simulink model "sun_path_1"  (R2017a)
settings: Solver=FixedStepAuto  StartTime=1  StopTime=1  FixedStep=1  RelTol=1e-3
libraries: simulink_extras x5
settings Model: Creator=zhiangz  LastModifiedBy=zhiangz

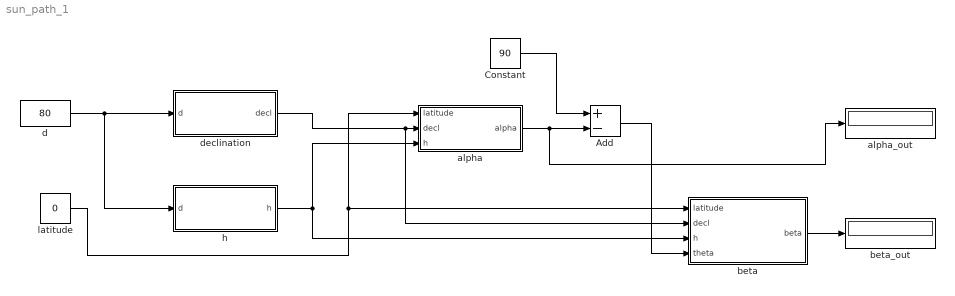
== system sun_path_1 ==
  Add : Sum  Inputs=+-
  Constant : Constant  Value=90
  alpha : Subsystem
  alpha_out : Display
  beta : Subsystem
  beta_out : Display
  d : Constant  Value=80
  declination : Subsystem
  h : Subsystem
  latitude : Constant  Value=0
  wires:
  alpha/1(alpha) -> alpha_out/1, Add/2
  Constant/1 -> Add/1
  Add/1 -> beta/4(theta)
  d/1 -> h/1(d), declination/1(d)
  latitude/1 -> alpha/1(latitude), beta/1(latitude)
  declination/1(decl) -> beta/2(decl), alpha/2(decl)
  h/1(h) -> alpha/3(h), beta/3(h)
  beta/1(beta) -> beta_out/1

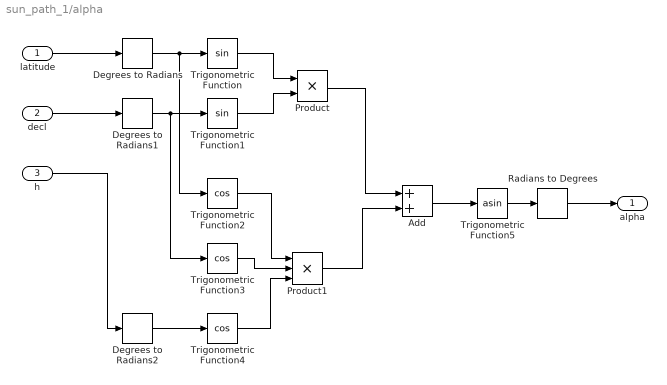
== system sun_path_1/alpha ==
  latitude : Inport
  decl : Inport  Port=2
  h : Inport  Port=3
  Add : Sum
  Degrees to Radians : simulink_extras/Transformations/Degrees to Radians
  Degrees to Radians1 : simulink_extras/Transformations/Degrees to Radians
  Degrees to Radians2 : simulink_extras/Transformations/Degrees to Radians
  Product : Product
  Product1 : Product  Inputs=3
  Radians to Degrees : simulink_extras/Transformations/Radians to Degrees
  Trigonometric Function : Trigonometry
  Trigonometric Function1 : Trigonometry
  Trigonometric Function2 : Trigonometry  Operator=cos
  Trigonometric Function3 : Trigonometry  Operator=cos
  Trigonometric Function4 : Trigonometry  Operator=cos
  Trigonometric Function5 : Trigonometry  Operator=asin
  alpha : Outport
  wires:
  latitude/1 -> Degrees to Radians/1
  Degrees to Radians/1 -> Trigonometric Function2/1, Trigonometric Function/1
  decl/1 -> Degrees to Radians1/1
  Degrees to Radians1/1 -> Trigonometric Function3/1, Trigonometric Function1/1
  Trigonometric Function/1 -> Product/1
  Trigonometric Function1/1 -> Product/2
  h/1 -> Degrees to Radians2/1
  Trigonometric Function2/1 -> Product1/1
  Trigonometric Function3/1 -> Product1/2
  Trigonometric Function4/1 -> Product1/3
  Product/1 -> Add/1
  Product1/1 -> Add/2
  Add/1 -> Trigonometric Function5/1
  Trigonometric Function5/1 -> Radians to Degrees/1
  Radians to Degrees/1 -> alpha/1
  Degrees to Radians2/1 -> Trigonometric Function4/1

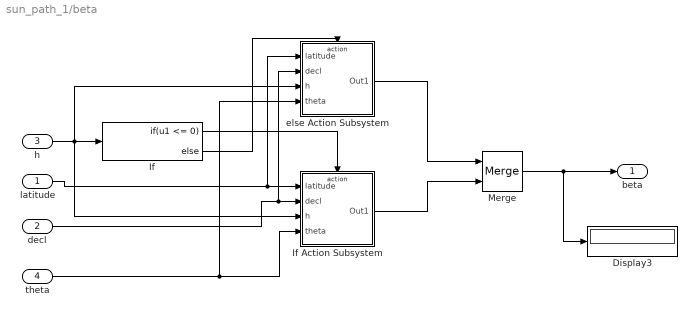
== system sun_path_1/beta ==
  latitude : Inport
  decl : Inport  Port=2
  h : Inport  Port=3
  theta : Inport  Port=4
  Display3 : Display
  If : If  IfExpression=u1 <= 0
  If Action Subsystem : Subsystem  TreatAsAtomicUnit=on
  Merge : Merge
  else Action Subsystem : Subsystem  TreatAsAtomicUnit=on
  beta : Outport
  wires:
  h/1 -> else Action Subsystem/3(h), If Action Subsystem/3(h), If/1
  If/1 -> If Action Subsystem/Action
  latitude/1 -> else Action Subsystem/1(latitude), If Action Subsystem/1(latitude)
  decl/1 -> else Action Subsystem/2(decl), If Action Subsystem/2(decl)
  theta/1 -> else Action Subsystem/4(theta), If Action Subsystem/4(theta)
  If/2 -> else Action Subsystem/Action
  Merge/1 -> Display3/1, beta/1
  else Action Subsystem/1(Out1) -> Merge/1
  If Action Subsystem/1(Out1) -> Merge/2

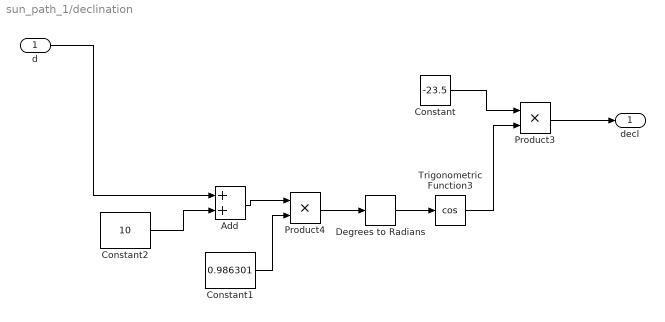
== system sun_path_1/declination ==
  d : Inport
  Add : Sum
  Constant : Constant  Value=-23.5
  Constant1 : Constant  Value=0.986301
  Constant2 : Constant  Value=10
  Degrees to Radians : simulink_extras/Transformations/Degrees to Radians
  Product3 : Product
  Product4 : Product
  Trigonometric Function3 : Trigonometry  Operator=cos
  decl : Outport
  wires:
  Trigonometric Function3/1 -> Product3/2
  Constant1/1 -> Product4/2
  Constant/1 -> Product3/1
  Product4/1 -> Degrees to Radians/1
  Add/1 -> Product4/1
  d/1 -> Add/1
  Constant2/1 -> Add/2
  Product3/1 -> decl/1
  Degrees to Radians/1 -> Trigonometric Function3/1

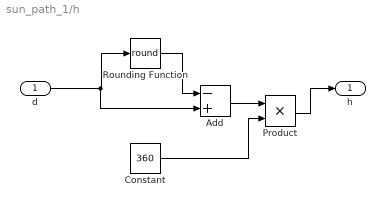
== system sun_path_1/h ==
  d : Inport
  Add : Sum  Inputs=-+
  Constant : Constant  Value=360
  Product : Product
  Rounding Function : Rounding  Operator=round
  h : Outport
  wires:
  d/1 -> Add/2, Rounding Function/1
  Rounding Function/1 -> Add/1
  Add/1 -> Product/1
  Constant/1 -> Product/2
  Product/1 -> h/1

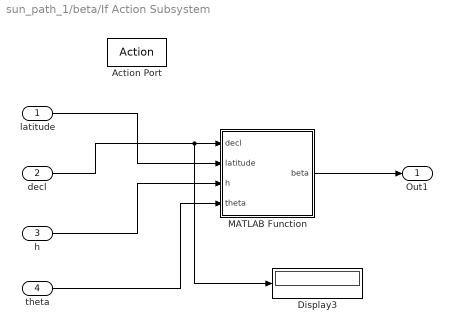
== system sun_path_1/beta/If Action Subsystem ==
  latitude : Inport
  decl : Inport  Port=2
  h : Inport  Port=3
  theta : Inport  Port=4
  Action Port : ActionPort  ActionType=then
  Display3 : Display
  MATLAB Function : MATLAB Function  TreatAsAtomicUnit=on
  Out1 : Outport
  wires:
  MATLAB Function/1(beta) -> Out1/1
  latitude/1 -> MATLAB Function/2(latitude)
  decl/1 -> Display3/1, MATLAB Function/1(decl)
  h/1 -> MATLAB Function/3(h)
  theta/1 -> MATLAB Function/4(theta)

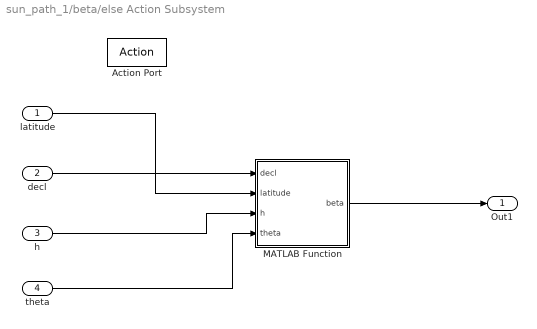
== system sun_path_1/beta/else Action Subsystem ==
  latitude : Inport
  decl : Inport  Port=2
  h : Inport  Port=3
  theta : Inport  Port=4
  Action Port : ActionPort  ActionType=else
  MATLAB Function : MATLAB Function  TreatAsAtomicUnit=on
  Out1 : Outport
  wires:
  decl/1 -> MATLAB Function/1(decl)
  latitude/1 -> MATLAB Function/2(latitude)
  h/1 -> MATLAB Function/3(h)
  theta/1 -> MATLAB Function/4(theta)
  MATLAB Function/1(beta) -> Out1/1

== matlab function sun_path_1/beta/If Action Subsystem/MATLAB Function ==
  data: decl input; beta output; latitude input; h input; theta input
function beta = beta_2(decl, latitude, h, theta)
decl = deg2rad(decl);
latitude = deg2rad(latitude);
h = deg2rad(h);
theta = deg2rad(theta);
trian_val = (sin(decl)*cos(latitude) - cos(h)*cos(decl)...
            *sin(latitude))/sin(theta);
trian_val = min(max(trian_val, -1), 1);
beta = -acos(trian_val);
beta = rad2deg(beta);
end

== matlab function sun_path_1/beta/else Action Subsystem/MATLAB Function ==
  data: decl input; beta output; latitude input; h input; theta input
function beta = beta_1(decl, latitude, h, theta)
decl = deg2rad(decl);
latitude = deg2rad(latitude);
h = deg2rad(h);
theta = deg2rad(theta);
trian_val = (sin(decl)*cos(latitude) - cos(h)*cos(decl)...
            *sin(latitude))/sin(theta);
trian_val = min(max(trian_val, -1), 1);
beta = acos(trian_val);
beta = rad2deg(beta);
end
